simulink subsystem "physics_sim"  (R2022a)
settings: Solver=VariableStepAuto  StartTime=0.0  StopTime=10.0  RelTol=1e-3
settings Model: Creator=Jon  LastModifiedBy=Jon

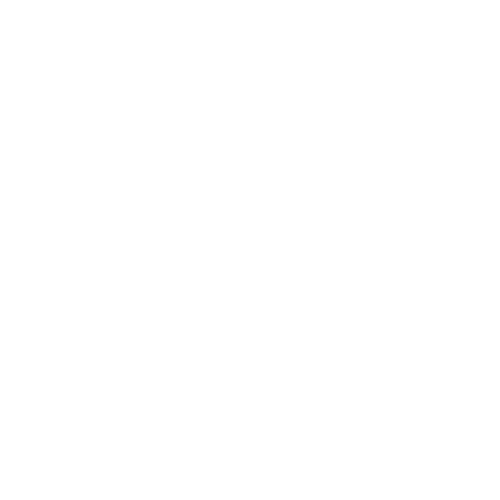
[thumbnail: Simulink's stored preview of the top-level diagram]
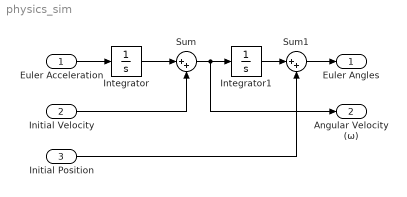
== system physics_sim ==
  Euler Acceleration : Inport
  Initial Velocity : Inport  Port=2
  Initial Position : Inport  Port=3
  Integrator : Integrator
  Integrator1 : Integrator
  Sum : Sum  Inputs=|++
  Sum1 : Sum  Inputs=|++
  Euler Angles : Outport
  Angular Velocity (ω) : Outport  Port=2
  wires:
  Euler Acceleration/1 -> Integrator/1
  Integrator/1 -> Sum/1
  Initial Velocity/1 -> Sum/2
  Sum/1 -> Integrator1/1, Angular Velocity (ω)/1
  Integrator1/1 -> Sum1/1
  Sum1/1 -> Euler Angles/1
  Initial Position/1 -> Sum1/2
